simulink model "nonlinear_spacecraft_quaternion_earth_ponting"  (R2015b)
settings: Solver=VariableStepAuto  StartTime=0.0  StopTime=stop_time  RelTol=1e-6
undefined symbols (not defined in the file): B_quaternion, J_x, J_y, J_z, K_d, K_p, n, x_0
settings Model: Creator=Krunal's PC  LastModifiedBy=Krunal's PC

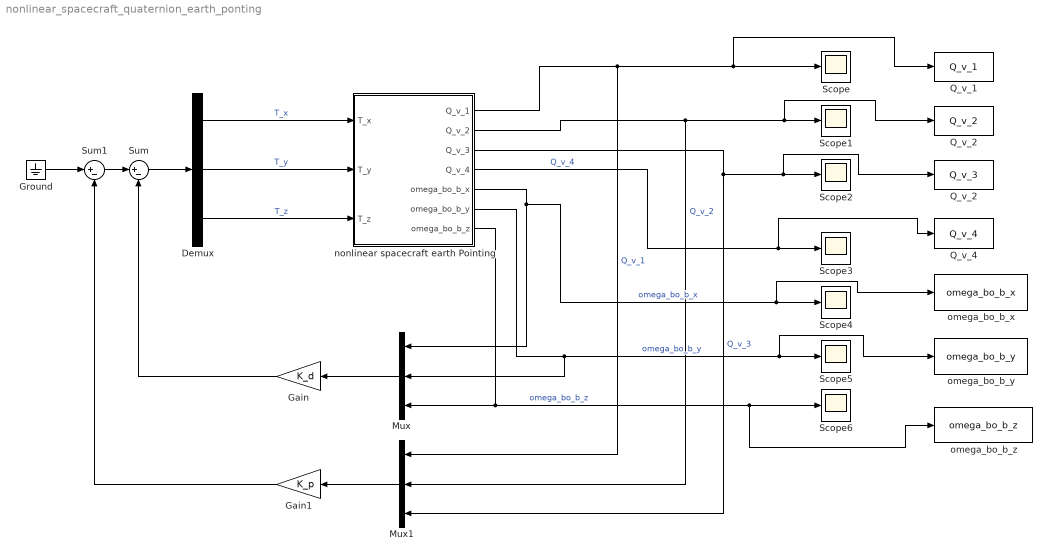
== system nonlinear_spacecraft_quaternion_earth_ponting ==
  " Q_v_2" : ToWorkspace  VariableName=Q_v_3  SampleTime=-1
  Demux : Demux  Outputs=3
  Gain : Gain  Gain=K_d
  Gain1 : Gain  Gain=K_p
  Ground : Ground
  Mux : Mux  Inputs=3
  Mux1 : Mux  Inputs=3
  Q_v_1 : ToWorkspace  VariableName=Q_v_1  SampleTime=-1
  Q_v_2 : ToWorkspace  VariableName=Q_v_2  SampleTime=-1
  Q_v_4 : ToWorkspace  VariableName=Q_v_4  SampleTime=-1
  Scope{,1..6} (7 alike) : Scope
  Sum : Sum  Inputs=|+-
  Sum1 : Sum  Inputs=|+-
  nonlinear spacecraft earth Pointing : Subsystem
  omega_bo_b_x : ToWorkspace  VariableName=omega_bo_b_x  SampleTime=-1
  omega_bo_b_y : ToWorkspace  VariableName=omega_bo_b_y  SampleTime=-1
  omega_bo_b_z : ToWorkspace  VariableName=omega_bo_b_z  SampleTime=-1
  wires:
  Demux/1 -> nonlinear spacecraft earth Pointing/1(T_x)  "T_x"
  Demux/2 -> nonlinear spacecraft earth Pointing/2(T_y)  "T_y"
  Demux/3 -> nonlinear spacecraft earth Pointing/3(T_z)  "T_z"
  nonlinear spacecraft earth Pointing/1(Q_v_1) -> Mux1/1, Q_v_1/1, Scope/1  "Q_v_1"
  nonlinear spacecraft earth Pointing/2(Q_v_2) -> Q_v_2/1, Scope1/1, Mux1/2  "Q_v_2"
  nonlinear spacecraft earth Pointing/3(Q_v_3) -> Mux1/3, " Q_v_2"/1, Scope2/1  "Q_v_3"
  nonlinear spacecraft earth Pointing/4(Q_v_4) -> Q_v_4/1, Scope3/1  "Q_v_4"
  nonlinear spacecraft earth Pointing/5(omega_bo_b_x) -> Mux/1, omega_bo_b_x/1, Scope4/1  "omega_bo_b_x"
  nonlinear spacecraft earth Pointing/6(omega_bo_b_y) -> Mux/2, omega_bo_b_y/1, Scope5/1  "omega_bo_b_y"
  nonlinear spacecraft earth Pointing/7(omega_bo_b_z) -> Mux/3, omega_bo_b_z/1, Scope6/1  "omega_bo_b_z"
  Mux/1 -> Gain/1
  Mux1/1 -> Gain1/1
  Gain/1 -> Sum/2
  Sum/1 -> Demux/1
  Sum1/1 -> Sum/1
  Gain1/1 -> Sum1/2
  Ground/1 -> Sum1/1

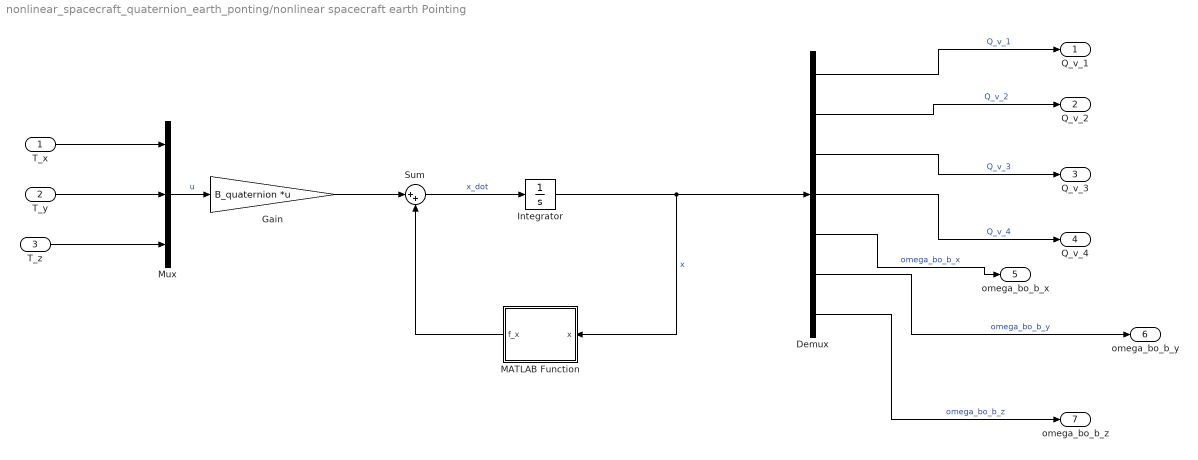
== system nonlinear_spacecraft_quaternion_earth_ponting/nonlinear spacecraft earth Pointing ==
  T_x : Inport
  T_y : Inport  Port=2
  T_z : Inport  Port=3
  Demux : Demux  Outputs=7
  Gain : Gain  Gain=B_quaternion  Multiplication=Matrix(K*u)
  Integrator : Integrator  InitialCondition=x_0
  MATLAB Function : MATLAB Function  TreatAsAtomicUnit=on
  Mux : Mux  Inputs=3
  Sum : Sum  Inputs=|++
  Q_v_1 : Outport
  Q_v_2 : Outport  Port=2
  Q_v_3 : Outport  Port=3
  Q_v_4 : Outport  Port=4
  omega_bo_b_x : Outport  Port=5
  omega_bo_b_y : Outport  Port=6
  omega_bo_b_z : Outport  Port=7
  wires:
  T_z/1 -> Mux/3
  Integrator/1 -> MATLAB Function/1(x), Demux/1  "x"
  T_y/1 -> Mux/2
  T_x/1 -> Mux/1
  Mux/1 -> Gain/1  "u"
  Gain/1 -> Sum/1
  Sum/1 -> Integrator/1  "x_dot"
  MATLAB Function/1(f_x) -> Sum/2
  Demux/1 -> Q_v_1/1  "Q_v_1"
  Demux/2 -> Q_v_2/1  "Q_v_2"
  Demux/3 -> Q_v_3/1  "Q_v_3"
  Demux/4 -> Q_v_4/1  "Q_v_4"
  Demux/5 -> omega_bo_b_x/1  "omega_bo_b_x"
  Demux/6 -> omega_bo_b_y/1  "omega_bo_b_y"
  Demux/7 -> omega_bo_b_z/1  "omega_bo_b_z"

== matlab function nonlinear_spacecraft_quaternion_earth_ponting/nonlinear spacecraft earth Pointing/MATLAB Function ==
  data: x input; f_x output; J_x parameter; J_y parameter; J_z parameter; n parameter
function f_x = fcn(x,J_x,J_y,J_z,n)
Q_v=zeros(3,1);
omega_bo_b=zeros(3,1);
Q_v(1,1)=x(1);
Q_v(2,1)=x(2);
Q_v(3,1)=x(3);
Q_4=x(4);
omega_bo_b(1,1)=x(5);
omega_bo_b(2,1)=x(6);
omega_bo_b(3,1)=x(7);
  
J = [J_x 0 0; 0 J_y 0; 0 0 J_z];
Q_v_dot=1/2*(Q_4*eye(3)+cross_operator(Q_v))*omega_bo_b;           
Q_4_dot= -1/2*Q_v'*omega_bo_b;
omega_oi_o=[0; -n; 0];

C_Q= (Q_4^2-Q_v'*Q_v)*eye(3)+2*Q_v*Q_v'-2*Q_4*cross_operator(Q_v);


omega_bo_b_dot_1=inv(J)*((-J*cross_operator(C_Q*omega_oi_o)-cross_operator(omega_bo_b)*J+cross_operator(J*C_Q*omega_oi_o)-cross_operator(C_Q*omega_oi_o)*J)*omega_bo_b-(cross_operator(C_Q*omega_oi_o)*J*C_Q*omega_oi_o));


f_x=zeros(7,1);

f_x(1,1)= Q_v_dot(1,1);
f_x(2,1)= Q_v_dot(2,1);
f_x(3,1)= Q_v_dot(3,1);
f_x(4,1)=Q_4_dot;
f_x(5,1)= omega_bo_b_dot_1(1,1);
f_x(6,1)= omega_bo_b_dot_1(2,1);
f_x(7,1)= omega_bo_b_dot_1(3,1);
end

 function v_cross = cross_operator(v)

v_cross=[0 -v(3) v(2);
         v(3) 0 -v(1);
         -v(2) v(1) 0];

end
